simulink model "sim"  (R2018a)
settings: Solver=VariableStepAuto  StartTime=0.0  StopTime=10.0  RelTol=1e-3
values from neighbouring files (symbols this model uses):
  b = 0.2    [sol.m]
  g = 9.8    [sol.m]
  I = 0.006    [sol.m]
  l = 0.3    [sol.m]
  M = 0.7    [sol.m]
  m = 0.8    [sol.m]
undefined symbols (not defined in the file or in its folder): magnitude
settings Model: Creator=daniel  LastModifiedBy=daniel

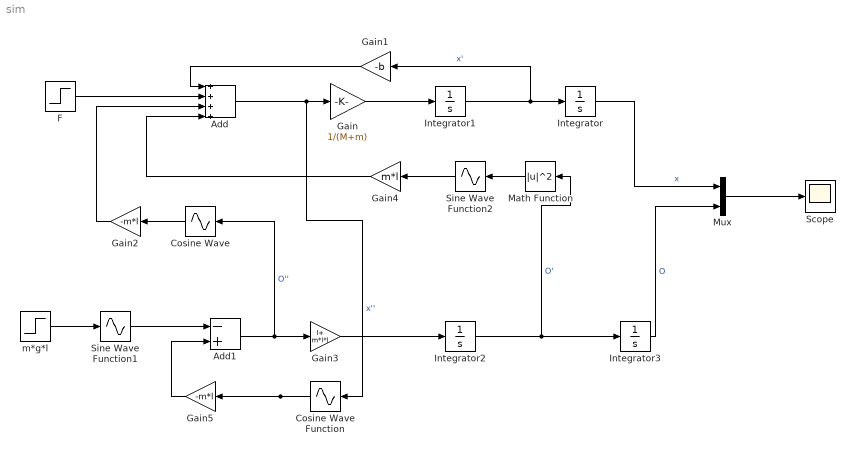
== system sim ==
  Add : Sum  Inputs=++++
  Add1 : Sum  Inputs=-+
  "Cosine Wave " : Sin  TimeSource=Use external signal  Bias=pi  SampleTime=0
  Cosine Wave Function : Sin  TimeSource=Use external signal  Bias=pi  SampleTime=0
  "F " : Step  SampleTime=0
  Gain : Gain  Gain=1/(M+m)
  Gain1 : Gain  Gain=-b
  Gain2 : Gain  Gain=-m*l
  Gain3 : Gain  Gain=I+ m*l*l
  Gain4 : Gain  Gain=m*l
  Gain5 : Gain  Gain=-m*l
  Integrator : Integrator
  Integrator1 : Integrator
  Integrator2 : Integrator
  Integrator3 : Integrator  InitialCondition=0.01
  Math Function : Math  Operator=magnitude^2  SaturateOnIntegerOverflow=on
  Mux : Mux  Inputs=2
  Scope : Scope
  Sine Wave Function1 : Sin  TimeSource=Use external signal  SampleTime=0
  Sine Wave Function2 : Sin  TimeSource=Use external signal  SampleTime=0
  m*g*l : Step  Time=m*g*l  SampleTime=0
  wires:
  Add/1 -> Cosine Wave Function/1, Gain/1  "x''"
  Gain/1 -> Integrator1/1
  Integrator1/1 -> Gain1/1, Integrator/1  "x'"
  "Cosine Wave "/1 -> Gain2/1
  Integrator/1 -> Mux/1  "x"
  Mux/1 -> Scope/1
  Integrator2/1 -> Math Function/1, Integrator3/1  "O'"
  Add1/1 -> "Cosine Wave "/1, Gain3/1  "O''"
  Gain3/1 -> Integrator2/1
  Sine Wave Function1/1 -> Add1/1
  Cosine Wave Function/1 -> Gain5/1
  Gain5/1 -> Add1/2
  m*g*l/1 -> Sine Wave Function1/1
  Integrator3/1 -> Mux/2  "O"
  "F "/1 -> Add/2
  Gain1/1 -> Add/1
  Gain2/1 -> Add/3
  Gain4/1 -> Add/4
  Sine Wave Function2/1 -> Gain4/1
  Math Function/1 -> Sine Wave Function2/1
